simulink model "wecModel_Morrison_Heave_091514"  (R2014a)
settings: Solver=ode4  StartTime=0  StopTime=200  FixedStep=0.05  RelTol=1e-3
undefined symbols (not defined in the file): body, constraint, simu, waves, X, Y, Z
libraries: nesl_utility x18, vrlib x8, sm_lib x7, WECSim_Lib x2
(part 1 of 2)
settings Model: Creator=mlawson  LastModifiedBy=ntom
settings SolverCC: AlgebraicLoopSolver=LineSearch
settings DataIOCC: LimitDataPoints=off  SaveOutput=off  SaveTime=off
settings DebuggingCC: UnderspecifiedInitializationDetection=Classic  StateNameClashWarn=warning
settings ExplorerConfigSet: InternalSimMechanicsExplorerSettings="<ExplorerConfiguration><canonicalview>default</canonicalview><TilePanel><TileInfo><Tiles Columns=\"1\" Count=\"1\" Rows=\"1\"><Column Left=\"2\" Weight=\"1\"/><Column Left=\"1335\"/><Row Top=\"2\" Weight=\"1\"/><Row Top=\"911\"/><Tile Height=\"1\" Width=\"1\" X=\"0\" Y=\"0\"/></Tiles></TileInfo><SceneInfo><SceneViewer><BGColor><R>0.60000002384185791</R><G>0.60000002384185791</G><B>0.60000002384185791</B></BGColor><Camera><Position><X>365.37645888990272</X><Y>-369.82486814446582</Y><Z>359.64809521743916</Z></Position><Center><X>-6.7351450971904585</X><Y>2.2867358426280204</Y><Z>-12.463508769654169</Z></Center><Up><X>-0.40824829046386307</X><Y>0.40824829046386307</Y><Z>0.81649658092772615</Z></Up><Left>-57.820127362122818</Left><Right>57.820127362122818</Right><Bottom>-38.308817187253304</Bottom><Top>38.308817187253304</Top></Camera></SceneViewer></SceneInfo></TilePanel></ExplorerConfiguration>"

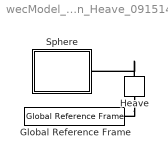
== system wecModel_Morrison_Heave_091514 ==
  Global Reference Frame : WECSim_Lib/Frames/Global Reference Frame  waves=waves  simu=simu
  Heave : WECSim_Lib/Constraints/Heave  constraint=constraint(1)
      settings: AttributesFormatString=%<constraint>
  Sphere : Subsystem  AncestorBlock=WECSim_Lib/Body Elements/Rigid Body  mask(BodyElements){body=body(1)}
      mask prompts: body "Body Name:"
      mask help: This block represents a rigid body. The variable name input below must be 'body(i)' where i=1,2,...
      mask init:
      | if exist('body','var')
      |     h=[gcb '/Structure/Body Properties'];
      |     geomFile=body.geom.file;
      |     set_param(h,'ExtGeomFileName',geomFile);
      |     h=[gcb '/To Workspace'];
      |     responseName=[body.name '_out'];
      |     set_param(h,'VariableName',responseName);
      | end
      | clear bc h geomFile responseName
      settings: AttributesFormatString=%<body>
  connections:
  Heave/RConn1 -- Sphere/RConn1
  Heave/LConn1 -- Global Reference Frame/RConn1

== system wecModel_Morrison_Heave_091514/Sphere ==
  Bus Creator : BusCreator  Inputs=5
  Bus Creator1 : BusCreator  Inputs=3
  Bus Selector : BusSelector  OutputSignals=disp,vel,accel
  Bus Selector1 : BusSelector  OutputSignals=F_Excitation,F_Restoring,F_Viscous,F_Mooring,F_Radiation
  Hydrostatic Restoring Force Calculation : Subsystem
  Mooring Force Calculation (Map) : Subsystem
  Structure : Subsystem
  Sum : Sum  Inputs=+----
  To Workspace : ToWorkspace  VariableName=Sphere_out  SaveFormat=Structure With Time  SampleTime=-1
  ViscousDampingForceCalculation : Subsystem
  Wave Diffraction and Excitation Force Calculation : Subsystem
  Wave Radiation Forces Calculation : Subsystem
  Conn : PMIOPort  Port=1  Side=Right
  wires:
  Bus Selector1/5 -> Sum/5  "<F_Radiation>"
  Bus Selector1/4 -> Sum/4  "<F_Mooring>"
  Bus Selector1/3 -> Sum/3  "<F_Viscous>"
  Bus Selector1/2 -> Sum/2  "<F_Restoring>"
  Bus Selector1/1 -> Sum/1  "<F_Excitation>"
  Wave Diffraction and Excitation Force Calculation/1(F_Excitation) -> Bus Creator/1
  Wave Radiation Forces Calculation/1(F_Radiation) -> Bus Creator/2
  Hydrostatic Restoring Force Calculation/1(F_Restoring) -> Bus Creator/3
  ViscousDampingForceCalculation/1(F_Viscous) -> Bus Creator/4
  Mooring Force Calculation (Map)/1(F_Mooring) -> Bus Creator/5
  Bus Selector/3 -> ViscousDampingForceCalculation/3(Acceleration), Wave Radiation Forces Calculation/2(Acceleration)  "<accel>"
  Bus Creator1/1 -> To Workspace/1
  Bus Creator/1 -> Bus Selector1/1, Bus Creator1/3
  Structure/1(Response) -> Bus Creator1/1, Bus Selector/1
  Bus Selector/2 -> Wave Radiation Forces Calculation/1(Velocity), Mooring Force Calculation (Map)/2(Velocity), ViscousDampingForceCalculation/1(Velocity)  "<vel>"
  Bus Selector/1 -> Hydrostatic Restoring Force Calculation/1(Displacement), Mooring Force Calculation (Map)/1(Displacement), ViscousDampingForceCalculation/2(Displacement)  "<disp>"
  Sum/1 -> Structure/1(F_vector), Bus Creator1/2
  connections:
  Structure/RConn1 -- Conn/RConn1

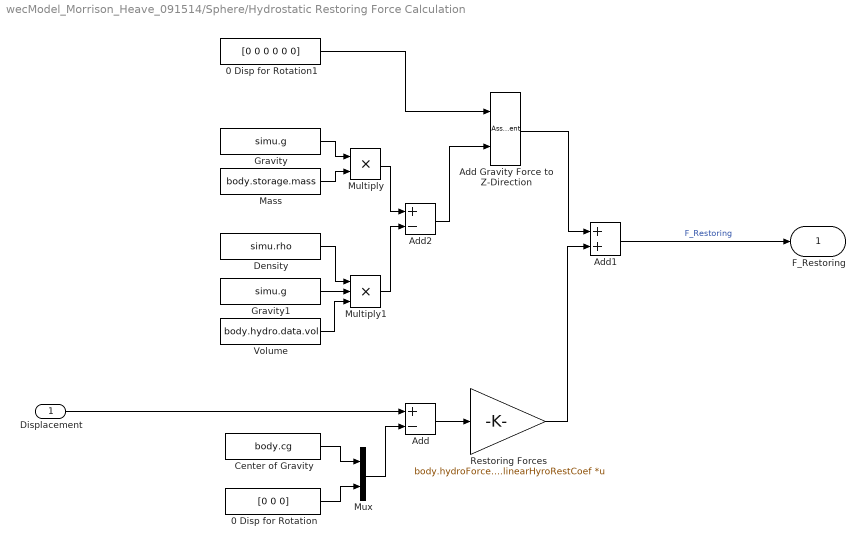
== system wecModel_Morrison_Heave_091514/Sphere/Hydrostatic Restoring Force Calculation ==
  Displacement : Inport
  0 Disp for Rotation : Constant  Value=[0 0 0]
  0 Disp for Rotation1 : Constant  Value=[0 0 0 0 0 0]
  Add : Sum  Inputs=+-
  Add Gravity Force to Z-Direction : Assignment  Indices=3
  Add1 : Sum
  Add2 : Sum  Inputs=+-
  Center of Gravity : Constant  Value=body.cg
  Density : Constant  Value=simu.rho
  Gravity : Constant  Value=simu.g
  Gravity1 : Constant  Value=simu.g
  Mass : Constant  Value=body.storage.mass
  Multiply : Product  Inputs=**
  Multiply1 : Product  Inputs=***
  Mux : Mux  Inputs=2
  Restoring Forces : Gain  Gain=body.hydroForce.linearHyroRestCoef  Multiplication=Matrix(K*u)
  Volume : Constant  Value=body.hydro.data.vol
  F_Restoring : Outport
  wires:
  Restoring Forces/1 -> Add1/2
  Add2/1 -> Add Gravity Force to Z-Direction/2
  Multiply1/1 -> Add2/2
  Multiply/1 -> Add2/1
  Density/1 -> Multiply1/1
  Gravity1/1 -> Multiply1/2
  Volume/1 -> Multiply1/3
  Add1/1 -> F_Restoring/1  "F_Restoring"
  Add Gravity Force to Z-Direction/1 -> Add1/1
  0 Disp for Rotation1/1 -> Add Gravity Force to Z-Direction/1
  Mass/1 -> Multiply/2
  Gravity/1 -> Multiply/1
  0 Disp for Rotation/1 -> Mux/2
  Center of Gravity/1 -> Mux/1
  Mux/1 -> Add/2
  Displacement/1 -> Add/1
  Add/1 -> Restoring Forces/1

== system wecModel_Morrison_Heave_091514/Sphere/Mooring Force Calculation (Map) ==
  Displacement : Inport
  Velocity : Inport  Port=2
  0 Disp for Rotation : Constant  Value=[0 0 0]
  Add : Sum  Inputs=+-
  Center of Gravity : Constant  Value=body.cg
  Mooring Damping : Gain  Gain=body.mooring.c  Multiplication=Matrix(K*u)
  Mooring Stiffness : Gain  Gain=body.mooring.k  Multiplication=Matrix(K*u)
  Mooring Pre-Tension : Constant  Value=body.mooring.preTension
  Mux : Mux  Inputs=2
  sum : Sum  Inputs=++-
  F_Mooring : Outport
  wires:
  0 Disp for Rotation/1 -> Mux/2
  Center of Gravity/1 -> Mux/1
  Displacement/1 -> Add/1
  Mux/1 -> Add/2
  Add/1 -> Mooring Stiffness/1
  Mooring Pre-Tension/1 -> sum/3
  sum/1 -> F_Mooring/1  "F_Mooring"
  Mooring Damping/1 -> sum/2
  Velocity/1 -> Mooring Damping/1
  Mooring Stiffness/1 -> sum/1

== system wecModel_Morrison_Heave_091514/Sphere/Structure ==
  F_vector : Inport
  Body CG : sm_lib/Frames and Transforms/Reference Frame  BlockFunction=simmechanics.library.frames_transforms.reference_frame
  Body Properties : sm_lib/Body Elements/Solid  InertiaType=Custom  Mass=body.mass  MassUnits=kg  CenterOfMass=[0 0 0]  CenterOfMassUnits=m  MomentsOfInertia=body.momOfInertia  MomentsOfInertiaUnits=kg*m^2  ProductsOfInertia=[0 0 0]  ProductsOfInertiaUnits=kg*m^2  DensityBased=on  Density=1000  DensityUnits=kg/(m^3)  GraphicType=FromGeometry  MarkerShape=Sphere  MarkerSize=10  MarkerSizeUnits=m  GraphicVisPropType=SimpleVisualProperties  GraphicDiffuseColor=[1 1 0]  GraphicSpecularColor=[0.5 0.5 0.5 1.0]  GraphicAmbientColor=[0.15 0.15 0.15 1.0]  GraphicEmissiveColor=[0.0 0.0 0.0 1.0]  GraphicShininess=75  GraphicOpacity=1  GeometryShape=FromFile  RectangleSize=[1 1]  RectangleSizeUnits=m  BrickDimensions=[1 1 1]  BrickDimensionUnits=m  CylinderRadius=1  CylinderRadiusUnits=m  CylinderLength=1  CylinderLengthUnits=m  SphereRadius=1  SphereRadiusUnits=m  EllipsoidRadii=[1 1 1]  EllipsoidRadiiUnits=m  ExtrusionCrossSection=[1 1; -1 1; -1 -1; 1 -1]  ExtrusionCrossSectionUnits=m  ExtrusionLength=1  ExtrusionLengthUnits=m  PolygonNumSides=3  PolygonOuterRadius=1  PolygonOuterRadiusUnits=m  ExtGeomFileType=STL  ExtGeomFileName=geometry/skewed_p4scaleZ_sphere_2m_neutral.stl  ExtGeomFileUnits=m  RevolutionCrossSection=[1 1; 1 -1; 2 -1; 2 1]  RevolutionCrossSectionUnits=m  RevolutionExtent=Full  RevolutionAngle=180  RevolutionAngleUnits=deg  BlockFunction=simmechanics.library.body_elements.solid
  Bus Creator : BusCreator  Inputs=3
  External Force and Torque : sm_lib/Forces and Torques/External Force and Torque  ForceResolutionFrame=World  EnableForceX=off  EnableForceY=off  EnableForceZ=off  EnableForce=on  TorqueResolutionFrame=World  EnableTorqueX=off  EnableTorqueY=off  EnableTorqueZ=off  EnableTorque=on  BlockFunction=simmechanics.library.forces_torques.external_force_torque
  Motion Sensor: Stucture Response : Subsystem
  Selector : Selector  InputPortWidth=6  Indices=[1:3]
  Selector1 : Selector  InputPortWidth=6  Indices=[4:6]
  Setup CG : sm_lib/Frames and Transforms/Rigid Transform  TranslationMethod=Cartesian  TranslationLengthUnit=m  TranslationStandardAxis=+Z  TranslationStandardOffset=0  TranslationCartesianOffset=body.cg  TranslationROffset=0  TranslationROffsetUnits=m  TranslationZOffset=0  TranslationZOffsetUnits=m  TranslationThetaOffset=0  TranslationThetaOffsetUnits=deg  RotationMethod=None  RotationAngleUnits=rad  RotationStandardAxis=+Y  RotationAngle=0.05  RotationArbitraryAxis=[0.57735026918962584 0.57735026918962584 0.57735026918962584]  FollAlignAxisA=+X  BaseAlignAxisA=+Y  FollAlignAxisB=+Y  BaseAlignAxisB=+Z  BlockFunction=simmechanics.library.frames_transforms.rigid_transform
  Setup Initial Disp : sm_lib/Frames and Transforms/Rigid Transform  TranslationMethod=Cartesian  TranslationLengthUnit=m  TranslationStandardAxis=+Z  TranslationStandardOffset=0  TranslationCartesianOffset=body.initLinDisp  TranslationROffset=0  TranslationROffsetUnits=m  TranslationZOffset=0  TranslationZOffsetUnits=m  TranslationThetaOffset=0  TranslationThetaOffsetUnits=deg  RotationMethod=ArbitraryAxis  RotationAngleUnits=rad  RotationStandardAxis=+Y  RotationAngle=body.initAngularDispAngle  RotationArbitraryAxis=body.initAngularDispAxis  FollAlignAxisA=+X  BaseAlignAxisA=+Y  FollAlignAxisB=+Y  BaseAlignAxisB=+Z  BlockFunction=simmechanics.library.frames_transforms.rigid_transform
  Simulink-PS Converter1 : nesl_utility/Simulink-PS Converter  PhysicalDomain=network_engine_domain  SubClassName=ps_input  LeftPortType=input  RightPortType=output  PseudoPeriodic=off  Frequencies=[]  NoiseDistribution=none  NoiseParameters=[]  Unit=1  AffineConversion=off  InputFiltering=off  SimscapeFilterOrder=1  InputFilterTimeConstant=0.001  UdotUserProvided=1
  Simulink-PS Converter2 : nesl_utility/Simulink-PS Converter  PhysicalDomain=network_engine_domain  SubClassName=ps_input  LeftPortType=input  RightPortType=output  PseudoPeriodic=off  Frequencies=[]  NoiseDistribution=none  NoiseParameters=[]  Unit=1  AffineConversion=off  InputFiltering=off  SimscapeFilterOrder=1  InputFilterTimeConstant=0.001  UdotUserProvided=1
  World Frame : sm_lib/Frames and Transforms/World Frame  BlockFunction=simmechanics.library.frames_transforms.world_frame
  Connection(MFS) : PMIOPort  Port=1  Side=Right
  Response : Outport
  wires:
  Motion Sensor: Stucture Response/3(Acceleration) -> Bus Creator/3  "accel"
  Motion Sensor: Stucture Response/2(Velocity) -> Bus Creator/2  "vel"
  Motion Sensor: Stucture Response/1(Displacement) -> Bus Creator/1  "disp"
  Bus Creator/1 -> Response/1  "response"
  Selector1/1 -> Simulink-PS Converter2/1
  Selector/1 -> Simulink-PS Converter1/1
  F_vector/1 -> Selector/1, Selector1/1
  connections:
  Motion Sensor: Stucture Response/RConn1 -- Body CG/RConn1 -- External Force and Torque/RConn1 -- Body Properties/RConn1 -- Setup Initial Disp/RConn1
  World Frame/RConn1 -- Motion Sensor: Stucture Response/LConn1
  Setup Initial Disp/LConn1 -- Setup CG/RConn1
  Setup CG/LConn1 -- Connection(MFS)/RConn1
  Simulink-PS Converter2/RConn1 -- External Force and Torque/LConn2
  Simulink-PS Converter1/RConn1 -- External Force and Torque/LConn1

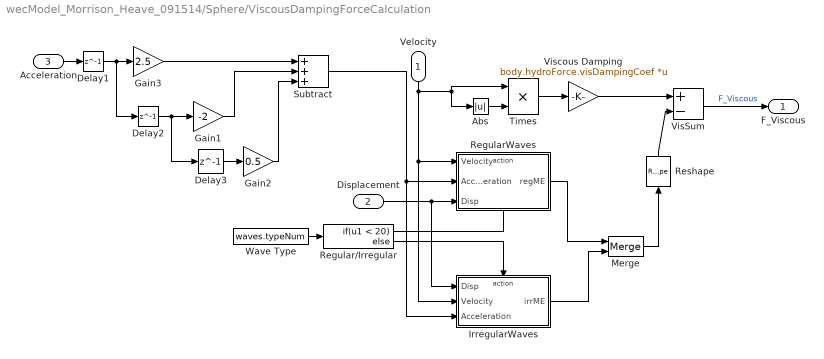
== system wecModel_Morrison_Heave_091514/Sphere/ViscousDampingForceCalculation ==
  Velocity : Inport
  Displacement : Inport  Port=2
  Acceleration : Inport  Port=3
  Abs : Abs
  Delay1 : Delay  DelayLength=1  InitialCondition=0
  Delay2 : Delay  DelayLength=1  InitialCondition=0
  Delay3 : Delay  DelayLength=1  InitialCondition=0
  Gain1 : Gain  Gain=-2
  Gain2 : Gain  Gain=0.5
  Gain3 : Gain  Gain=2.5
  IrregularWaves : Subsystem  TreatAsAtomicUnit=on
  Merge : Merge
  Regular/Irregular : If  IfExpression=u1 < 20
  RegularWaves : Subsystem  TreatAsAtomicUnit=on
  Reshape : Reshape
  Subtract : Sum  Inputs=+++
  Times : Product  Inputs=**
  "VisSum " : Sum  Inputs=+-
  Viscous Damping : Gain  Gain=body.hydroForce.visDampingCoef  Multiplication=Matrix(K*u)
  Wave Type : Constant  Value=waves.typeNum
  F_Viscous : Outport
  wires:
  Times/1 -> Viscous Damping/1
  Abs/1 -> Times/2
  Velocity/1 -> IrregularWaves/2(Velocity), RegularWaves/1(Velocity), Times/1, Abs/1
  Viscous Damping/1 -> "VisSum "/1
  "VisSum "/1 -> F_Viscous/1  "F_Viscous"
  Reshape/1 -> "VisSum "/2
  Wave Type/1 -> Regular/Irregular/1
  Regular/Irregular/2 -> IrregularWaves/Action
  Displacement/1 -> IrregularWaves/1(Disp), RegularWaves/3(Disp)
  Subtract/1 -> IrregularWaves/3(Acceleration), RegularWaves/2(Acceleration)
  Regular/Irregular/1 -> RegularWaves/Action
  IrregularWaves/1(irrME) -> Merge/2
  RegularWaves/1(regME) -> Merge/1
  Merge/1 -> Reshape/1
  Acceleration/1 -> Delay1/1
  Gain2/1 -> Subtract/3
  Gain1/1 -> Subtract/2
  Delay3/1 -> Gain2/1
  Delay2/1 -> Gain1/1, Delay3/1
  Delay1/1 -> Delay2/1, Gain3/1
  Gain3/1 -> Subtract/1

== system wecModel_Morrison_Heave_091514/Sphere/Wave Diffraction and Excitation Force Calculation ==
  Applied Ramp Function : Subsystem  TreatAsAtomicUnit=on
  If : If  IfExpression=u1 < 20
  If1 : If  NumInputs=2  IfExpression=u1 < u2
  Iregular Wave Excitation Force : Subsystem  TreatAsAtomicUnit=on
  Merge : Merge
  Merge1 : Merge
  No Ramp Function : Subsystem  TreatAsAtomicUnit=on
  Ramp Function Time : Constant  Value=simu.rampT
  Regular Wave Excitation Force : Subsystem  TreatAsAtomicUnit=on
  Wave Type : Constant  Value=waves.typeNum
  F_Excitation : Outport
  wires:
  Wave Type/1 -> If/1
  If/1 -> Regular Wave Excitation Force/Action
  If/2 -> Iregular Wave Excitation Force/Action
  Regular Wave Excitation Force/1(F_wave) -> Merge/1
  Iregular Wave Excitation Force/1(F_wave) -> Merge/2
  Ramp Function Time/1 -> If1/2
  Merge/1 -> No Ramp Function/1(In1), Applied Ramp Function/1(In1)
  If1/2 -> No Ramp Function/Action
  If1/1 -> Applied Ramp Function/Action
  Applied Ramp Function/1(Out1) -> Merge1/1
  No Ramp Function/1(Out1) -> Merge1/2
  Merge1/1 -> F_Excitation/1  "F_Excitation"
  [Clock] -> If1/1, Iregular Wave Excitation Force/1(Time)

== system wecModel_Morrison_Heave_091514/Sphere/Wave Radiation Forces Calculation ==
  Velocity : Inport
  Acceleration : Inport  Port=2
  Added Mass Forces : Gain  Gain=body.hydroForce.fAddedMass  Multiplication=Matrix(K*u)
  Damping Forces : Gain  Gain=body.hydroForce.fDamping  Multiplication=Matrix(K*u)
  Delay : Delay  DelayLength=1  InitialCondition=0
  Delay1 : Delay  DelayLength=1  InitialCondition=0
  Delay2 : Delay  DelayLength=1  InitialCondition=0
  Fluid Memory : MATLAB Function  TreatAsAtomicUnit=on
  Gain : Gain  Gain=2.5
  Gain1 : Gain  Gain=-2
  Gain2 : Gain  Gain=0.5
  Impulse Response Function K : Constant  Value=body.hydroForce.irkb
  Initial Zero Velocity : Constant  Value=simu.zeroVel
  Subtract : Sum  Inputs=+++
  Sum of Elements : Sum  Inputs=+++
  Time (relative to the current time step) : Constant  Value=simu.CTTime
  Wave Type : Constant  Value=waves.typeNum
  F_Radiation : Outport
  wires:
  Sum of Elements/1 -> F_Radiation/1  "F_Radiation"
  Gain2/1 -> Subtract/3
  Gain1/1 -> Subtract/2
  Delay2/1 -> Gain2/1
  Subtract/1 -> Added Mass Forces/1
  Delay1/1 -> Delay2/1, Gain1/1
  Gain/1 -> Subtract/1
  Delay/1 -> Gain/1, Delay1/1
  Acceleration/1 -> Delay/1
  Wave Type/1 -> Fluid Memory/1(check)
  Time (relative to the current time step)/1 -> Fluid Memory/5(CTTime)
  Impulse Response Function K/1 -> Fluid Memory/4(IRKB)
  Initial Zero Velocity/1 -> Fluid Memory/3(ZeroVel)
  Velocity/1 -> Damping Forces/1, Fluid Memory/2(v)
  Damping Forces/1 -> Sum of Elements/1  "F_Radiation Damping"
  Added Mass Forces/1 -> Sum of Elements/3  "F_Added Mass"
  Fluid Memory/1(F_FM) -> Sum of Elements/2  "F_Convolution Integral"

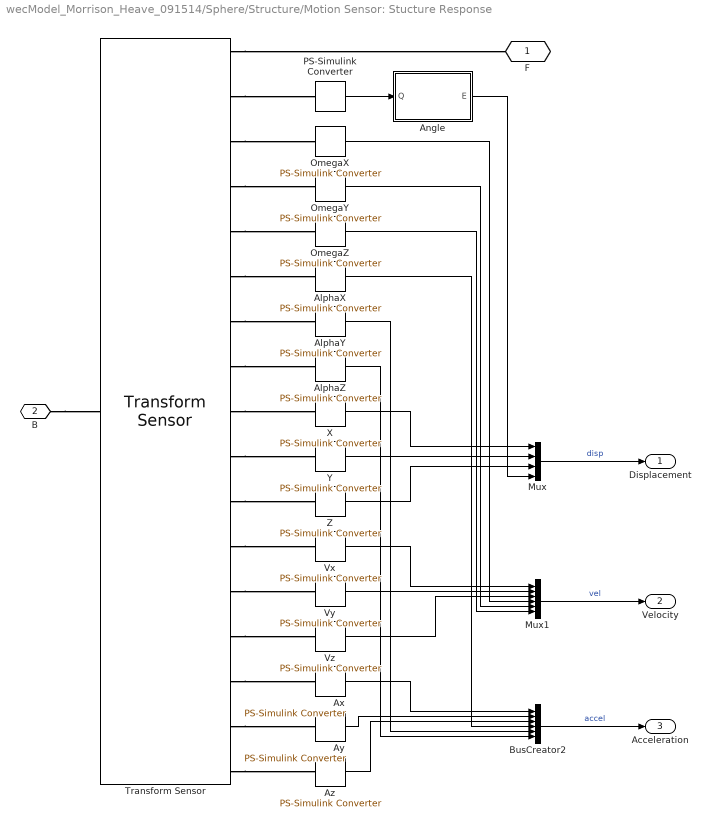
== system wecModel_Morrison_Heave_091514/Sphere/Structure/Motion Sensor: Stucture Response ==
  AlphaX : nesl_utility/PS-Simulink Converter  PhysicalDomain=network_engine_domain  SubClassName=ps_output  LeftPortType=input  RightPortType=output  PseudoPeriodic=off  Frequencies=[]  Unit=1  AffineConversion=off
  "AlphaY " : nesl_utility/PS-Simulink Converter  PhysicalDomain=network_engine_domain  SubClassName=ps_output  LeftPortType=input  RightPortType=output  PseudoPeriodic=off  Frequencies=[]  Unit=1  AffineConversion=off
  AlphaZ : nesl_utility/PS-Simulink Converter  PhysicalDomain=network_engine_domain  SubClassName=ps_output  LeftPortType=input  RightPortType=output  PseudoPeriodic=off  Frequencies=[]  Unit=1  AffineConversion=off
  Angle : MATLAB Function  TreatAsAtomicUnit=on
  Ax : nesl_utility/PS-Simulink Converter  PhysicalDomain=network_engine_domain  SubClassName=ps_output  LeftPortType=input  RightPortType=output  PseudoPeriodic=off  Frequencies=[]  Unit=1  AffineConversion=off
  Ay : nesl_utility/PS-Simulink Converter  PhysicalDomain=network_engine_domain  SubClassName=ps_output  LeftPortType=input  RightPortType=output  PseudoPeriodic=off  Frequencies=[]  Unit=1  AffineConversion=off
  Az : nesl_utility/PS-Simulink Converter  PhysicalDomain=network_engine_domain  SubClassName=ps_output  LeftPortType=input  RightPortType=output  PseudoPeriodic=off  Frequencies=[]  Unit=1  AffineConversion=off
  BusCreator2 : BusCreator  Inputs=6
  Mux : Mux
  Mux1 : Mux  Inputs=6
  OmegaX : nesl_utility/PS-Simulink Converter  PhysicalDomain=network_engine_domain  SubClassName=ps_output  LeftPortType=input  RightPortType=output  PseudoPeriodic=off  Frequencies=[]  Unit=1  AffineConversion=off
  OmegaY : nesl_utility/PS-Simulink Converter  PhysicalDomain=network_engine_domain  SubClassName=ps_output  LeftPortType=input  RightPortType=output  PseudoPeriodic=off  Frequencies=[]  Unit=1  AffineConversion=off
  OmegaZ : nesl_utility/PS-Simulink Converter  PhysicalDomain=network_engine_domain  SubClassName=ps_output  LeftPortType=input  RightPortType=output  PseudoPeriodic=off  Frequencies=[]  Unit=1  AffineConversion=off
  PS-Simulink Converter : nesl_utility/PS-Simulink Converter  PhysicalDomain=network_engine_domain  SubClassName=ps_output  LeftPortType=input  RightPortType=output  PseudoPeriodic=off  Frequencies=[]  Unit=1  AffineConversion=off
  Transform Sensor : sm_lib/Frames and Transforms/Transform Sensor  MeasurementFrame=World  SenseAngle=off  SenseAxis=off  SenseAngle1=off  SenseAngle2=off  SenseAngle3=off  SenseQ=on  SenseR=off  SenseOmegaX=on  SenseOmegaY=on  SenseOmegaZ=on  SenseOmega1=off  SenseOmega2=off  SenseOmega3=off  SenseQDot=off  SenseRDot=off  SenseAlphaX=on  SenseAlphaY=on  SenseAlphaZ=on  SenseAlpha1=off  SenseAlpha2=off  SenseAlpha3=off  SenseQDDot=off  SenseRDDot=off  SenseX=on  SenseY=on  SenseZ=on  SenseRad=off  SenseAzim=off  SenseDist=off  SenseInc=off  SenseXDot=on  SenseYDot=on  SenseZDot=on  SenseRadDot=off  SenseAzimDot=off  SenseDistDot=off  SenseIncDot=off  SenseXDDot=on  SenseYDDot=on  SenseZDDot=on  SenseRadDDot=off  SenseAzimDDot=off  SenseDistDDot=off  SenseIncDDot=off  BlockFunction=simmechanics.library.frames_transforms.transform_sensor
  Vx : nesl_utility/PS-Simulink Converter  PhysicalDomain=network_engine_domain  SubClassName=ps_output  LeftPortType=input  RightPortType=output  PseudoPeriodic=off  Frequencies=[]  Unit=1  AffineConversion=off
  Vy : nesl_utility/PS-Simulink Converter  PhysicalDomain=network_engine_domain  SubClassName=ps_output  LeftPortType=input  RightPortType=output  PseudoPeriodic=off  Frequencies=[]  Unit=1  AffineConversion=off
  Vz : nesl_utility/PS-Simulink Converter  PhysicalDomain=network_engine_domain  SubClassName=ps_output  LeftPortType=input  RightPortType=output  PseudoPeriodic=off  Frequencies=[]  Unit=1  AffineConversion=off
  X : nesl_utility/PS-Simulink Converter  PhysicalDomain=network_engine_domain  SubClassName=ps_output  LeftPortType=input  RightPortType=output  PseudoPeriodic=off  Frequencies=[]  Unit=1  AffineConversion=off
  Y : nesl_utility/PS-Simulink Converter  PhysicalDomain=network_engine_domain  SubClassName=ps_output  LeftPortType=input  RightPortType=output  PseudoPeriodic=off  Frequencies=[]  Unit=1  AffineConversion=off
  Z : nesl_utility/PS-Simulink Converter  PhysicalDomain=network_engine_domain  SubClassName=ps_output  LeftPortType=input  RightPortType=output  PseudoPeriodic=off  Frequencies=[]  Unit=1  AffineConversion=off
  F : PMIOPort  Port=1  Side=Right
  B : PMIOPort  Port=2  Side=Left
  Displacement : Outport
  Velocity : Outport  Port=2
  Acceleration : Outport  Port=3
  wires:
  OmegaZ/1 -> Mux1/6
  OmegaY/1 -> Mux1/5
  OmegaX/1 -> Mux1/4
  AlphaZ/1 -> BusCreator2/6
  "AlphaY "/1 -> BusCreator2/5
  Z/1 -> Mux/3
  Y/1 -> Mux/2
  X/1 -> Mux/1
  Angle/1(E) -> Mux/4
  BusCreator2/1 -> Acceleration/1  "accel"
  Mux1/1 -> Velocity/1  "vel"
  Mux/1 -> Displacement/1  "disp"
  Az/1 -> BusCreator2/3
  Ay/1 -> BusCreator2/2
  Ax/1 -> BusCreator2/1
  Vz/1 -> Mux1/3
  Vy/1 -> Mux1/2
  Vx/1 -> Mux1/1
  AlphaX/1 -> BusCreator2/4
  PS-Simulink Converter/1 -> Angle/1(Q)
  connections:
  Transform Sensor/RConn5 -- OmegaZ/LConn1
  Transform Sensor/RConn4 -- OmegaY/LConn1
  Transform Sensor/RConn3 -- OmegaX/LConn1
  Transform Sensor/RConn8 -- AlphaZ/LConn1
  Transform Sensor/RConn7 -- "AlphaY "/LConn1
  Transform Sensor/RConn6 -- AlphaX/LConn1
  Transform Sensor/RConn9 -- X/LConn1
  Transform Sensor/RConn10 -- Y/LConn1
  Transform Sensor/RConn11 -- Z/LConn1
  Transform Sensor/RConn12 -- Vx/LConn1
  Transform Sensor/RConn13 -- Vy/LConn1
  Transform Sensor/RConn14 -- Vz/LConn1
  Transform Sensor/RConn15 -- Ax/LConn1
  Transform Sensor/RConn16 -- Ay/LConn1
  Transform Sensor/RConn17 -- Az/LConn1
  Transform Sensor/RConn2 -- PS-Simulink Converter/LConn1
  B/RConn1 -- Transform Sensor/LConn1
  Transform Sensor/RConn1 -- F/RConn1

== system wecModel_Morrison_Heave_091514/Sphere/ViscousDampingForceCalculation/IrregularWaves ==
  Disp : Inport
  Velocity : Inport  Port=2
  Acceleration : Inport  Port=3
  Action Port : ActionPort
  Area : Constant  Value=body.characteristicAreaME  VectorParams1D=off
  Ca : Constant  Value=body.Ca  VectorParams1D=off
  Cd : Constant  Value=body.cdME  VectorParams1D=off
  MESum : Sum  Inputs=+  CollapseMode=Specified dimension
  MorrisonElements : Subsystem  TreatAsAtomicUnit=on
  Volume : Constant  Value=body.VME  VectorParams1D=off
  "r_{g}" : Constant  Value=body.rgME  VectorParams1D=off
  irrME : Outport
  wires:
  Velocity/1 -> MorrisonElements/2(Vel)
  "r_{g}"/1 -> MorrisonElements/1(r)
  Area/1 -> MorrisonElements/5(A)
  Cd/1 -> MorrisonElements/6(Cd)
  Disp/1 -> MorrisonElements/4(Disp)
  Acceleration/1 -> MorrisonElements/3(Accel)
  Volume/1 -> MorrisonElements/7(Vol)
  Ca/1 -> MorrisonElements/8(Ca)
  MorrisonElements/1(Force) -> MESum/1
  MESum/1 -> irrME/1

== system wecModel_Morrison_Heave_091514/Sphere/ViscousDampingForceCalculation/RegularWaves ==
  Velocity : Inport
  Acceleration : Inport  Port=2
  Disp : Inport  Port=3
  Action Port : ActionPort
  Area : Constant  Value=body.characteristicAreaME  VectorParams1D=off
  Ca : Constant  Value=body.Ca  VectorParams1D=off
  Cd : Constant  Value=body.cdME  VectorParams1D=off
  MESum : Sum  Inputs=+  CollapseMode=Specified dimension
  MorrisonElements : Subsystem  TreatAsAtomicUnit=on
  Volume : Constant  Value=body.VME  VectorParams1D=off
  "r_{g}" : Constant  Value=body.rgME  VectorParams1D=off
  regME : Outport
  wires:
  MESum/1 -> regME/1
  Velocity/1 -> MorrisonElements/2(Vel)
  "r_{g}"/1 -> MorrisonElements/1(r)
  Area/1 -> MorrisonElements/5(A)
  Cd/1 -> MorrisonElements/6(Cd)
  Disp/1 -> MorrisonElements/4(Disp)
  Acceleration/1 -> MorrisonElements/3(Accel)
  MorrisonElements/1(Force) -> MESum/1
  Volume/1 -> MorrisonElements/7(Vol)
  Ca/1 -> MorrisonElements/8(Ca)

== system wecModel_Morrison_Heave_091514/Sphere/Wave Diffraction and Excitation Force Calculation/Applied Ramp Function ==
  In1 : Inport
  Action Port : ActionPort
  Add : Sum
  Constant : Constant  Value=2
  Constant1 : Constant
  Divide : Product  Inputs=**/
  Sine Wave : Sin  Frequency=pi/simu.rampT  Phase=pi+pi/2  SampleTime=0
  Out1 : Outport
  wires:
  In1/1 -> Divide/1
  Divide/1 -> Out1/1
  Constant/1 -> Divide/3
  Constant1/1 -> Add/1
  Sine Wave/1 -> Add/2
  Add/1 -> Divide/2

== system wecModel_Morrison_Heave_091514/Sphere/Wave Diffraction and Excitation Force Calculation/Iregular Wave Excitation Force ==
  Time : Inport
  Action Port : ActionPort
  Excitation Re Part2 : Constant  Value=body.hydroForce.fExt.re  VectorParams1D=off
  Excitation Re Part3 : Constant  Value=body.hydroForce.fExt.im  VectorParams1D=off
  For Each Subsystem : Subsystem  TreatAsAtomicUnit=on
  Sum of Elements : Sum  Inputs=+  CollapseMode=Specified dimension
  dw1 : Constant  Value=(waves.w(end)-waves.w(1))/(waves.numFreq-1)  VectorParams1D=off
  wave frequency : Constant  Value=waves.w  VectorParams1D=off
  wave frequency1 : Constant  Value=waves.phaseRand'  VectorParams1D=off
  wave spectrum : Constant  Value=waves.A*2  VectorParams1D=off
  F_wave : Outport  PortDimensions=6
  wires:
  Excitation Re Part2/1 -> For Each Subsystem/3(wave fExt re)
  Excitation Re Part3/1 -> For Each Subsystem/4(wave fExt im)
  wave frequency/1 -> For Each Subsystem/2(wave freq)
  wave spectrum/1 -> For Each Subsystem/1(wave spectrum)
  For Each Subsystem/1(Out1) -> Sum of Elements/1
  Time/1 -> For Each Subsystem/5(Time)
  Sum of Elements/1 -> F_wave/1
  wave frequency1/1 -> For Each Subsystem/7(phaseRand)
  dw1/1 -> For Each Subsystem/6(dw)

== system wecModel_Morrison_Heave_091514/Sphere/Wave Diffraction and Excitation Force Calculation/No Ramp Function ==
  In1 : Inport
  Action Port : ActionPort
  Out1 : Outport
  wires:
  In1/1 -> Out1/1

== system wecModel_Morrison_Heave_091514/Sphere/Wave Diffraction and Excitation Force Calculation/Regular Wave Excitation Force ==
  Action Port : ActionPort
  Add : Sum  Inputs=+-
  Cos Wave : Sin  Amplitude=waves.A(1,:)  Frequency=waves.w(1,:)  Phase=pi/2  SampleTime=0
  Product : Product  Inputs=**
  Product1 : Product  Inputs=**
  Sin Wave : Sin  Amplitude=waves.A(1,:)  Frequency=waves.w(1,:)  SampleTime=0
  WAMIT Excitation Im Part : Constant  Value=body.hydroForce.fExt.im(1,:)  VectorParams1D=off
  WAMIT Excitation Re Part : Constant  Value=body.hydroForce.fExt.re(1,:)  VectorParams1D=off
  F_wave : Outport  PortDimensions=6
  wires:
  Cos Wave/1 -> Product/1
  WAMIT Excitation Re Part/1 -> Product/2
  Sin Wave/1 -> Product1/1
  Product1/1 -> Add/2
  WAMIT Excitation Im Part/1 -> Product1/2
  Product/1 -> Add/1
  Add/1 -> F_wave/1

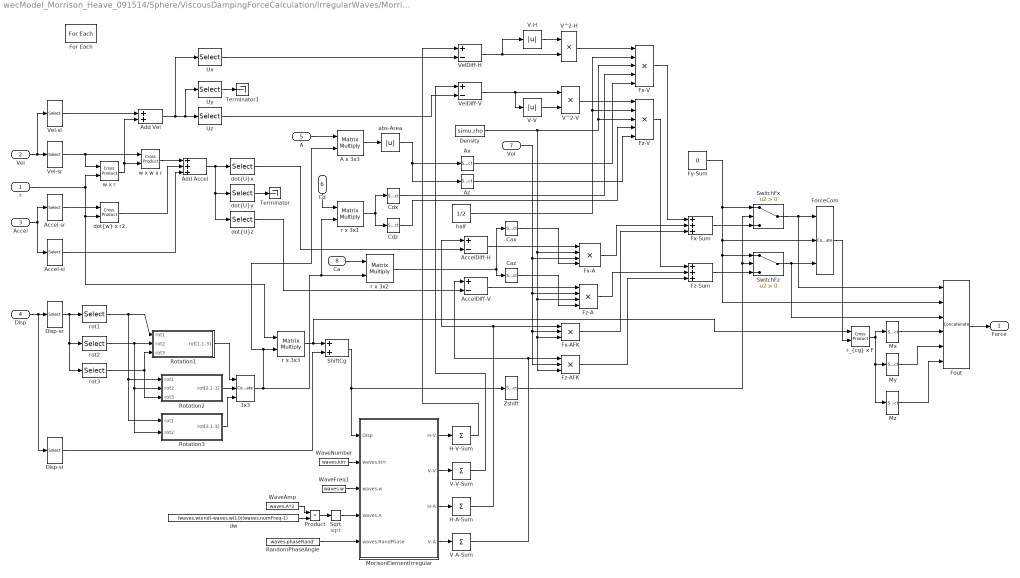
== system wecModel_Morrison_Heave_091514/Sphere/ViscousDampingForceCalculation/IrregularWaves/MorrisonElements ==
  r : Inport  Partition=on  PartitionDimension=1  PartitionWidth=1
  Vel : Inport  Port=2  Partition=off
  Accel : Inport  Port=3  Partition=off
  Disp : Inport  Port=4  Partition=off
  A : Inport  Port=5  Partition=on  PartitionDimension=1  PartitionWidth=1
  Cd : Inport  Port=6  Partition=on  PartitionDimension=1  PartitionWidth=1
  Vol : Inport  Port=7  Partition=on  PartitionDimension=1  PartitionWidth=1
  Ca : Inport  Port=8  Partition=on  PartitionDimension=1  PartitionWidth=1
  3x3 : Concatenate  NumInputs=3  Mode=Multidimensional array
  A x 3x3 : Product  Multiplication=Matrix(*)
  Accel-sl : Selector  InputPortWidth=6  Indices=[1 2 3]
  Accel-sr : Selector  InputPortWidth=6  Indices=[4 5 6]
  AccelDiff-H : Sum  Inputs=+-
  AccelDiff-V : Sum  Inputs=+-
  Add Accel : Sum  Inputs=+++
  Add Vel : Sum
  Ax : Selector  InputPortWidth=3  Indices=[1]
  Az : Selector  InputPortWidth=3  Indices=[3]
  Cax : Selector  InputPortWidth=3  Indices=[1]
  Caz : Selector  InputPortWidth=3  Indices=[3]
  Cdx : Selector  InputPortWidth=3  Indices=[1]
  Cdz : Selector  InputPortWidth=3  Indices=[3]
  Density : Constant  Value=simu.rho
  Disp-sl : Selector  InputPortWidth=6  Indices=[1 2 3]
  Disp-sr : Selector  InputPortWidth=6  Indices=[4 5 6]
  For Each : ForEach  DisableCoverage=on  IndexMode=One-based
  ForceCom : Concatenate  NumInputs=3  ConcatenateDimension=2
  Fout : Concatenate  NumInputs=6  Mode=Multidimensional array  ConcatenateDimension=2
  Fx-A : Product  Inputs=4
  Fx-AFK : Product  Inputs=3
  Fx-Sum : Sum  Inputs=+++
  Fx-V : Product  Inputs=5
  Fy-Sum : Constant  Value=0
  Fz-A : Product  Inputs=4
  Fz-AFK : Product  Inputs=3
  Fz-Sum : Sum  Inputs=+++
  Fz-V : Product  Inputs=5
  H-A-Sum : Sum  Inputs=+  CollapseMode=Specified dimension
  H-V-Sum : Sum  Inputs=+  CollapseMode=Specified dimension
  MorisonElementIrregular : Subsystem  TreatAsAtomicUnit=on
  Mx : Selector  InputPortWidth=3  Indices=[1]
  My : Selector  InputPortWidth=3  Indices=[2]
  Mz : Selector  InputPortWidth=3  Indices=[3]
  Product : Product
  RandomPhaseAngle : Constant  Value=waves.phaseRand'  VectorParams1D=off
  Rotation1 : Subsystem
  Rotation2 : Subsystem
  Rotation3 : Subsystem
  ShiftCg : Sum
  Sqrt : Sqrt  SaturateOnIntegerOverflow=on
  SwitchFx : Switch  Criteria=u2 > Threshold
  SwitchFz : Switch  Criteria=u2 > Threshold
  Terminator : Terminator
  Terminator1 : Terminator
  Ux : Selector  InputPortWidth=3  Indices=[1]
  Uy : Selector  InputPortWidth=3  Indices=[2]
  Uz : Selector  InputPortWidth=3  Indices=[3]
  V-A-Sum : Sum  Inputs=+  CollapseMode=Specified dimension
  V-H : Abs
  V-V : Abs
  V-V-Sum : Sum  Inputs=+  CollapseMode=Specified dimension
  V^2-H : Product
  V^2-V : Product
  Vel-sl : Selector  InputPortWidth=6  Indices=[1 2 3]
  "Vel-sr " : Selector  InputPortWidth=6  Indices=[4 5 6]
  VelDiff-H : Sum  Inputs=+-
  VelDiff-V : Sum  Inputs=+-
  WaveAmp : Constant  Value=waves.A*2  VectorParams1D=off
  WaveFreq1 : Constant  Value=waves.w  VectorParams1D=off
  WaveNumber : Constant  Value=waves.kirr  VectorParams1D=off
  Zshift : Selector  InputPortWidth=3  Indices=[3]
  abs-Area : Abs
  "dot{U}x" : Selector  InputPortWidth=3  Indices=[1]
  "dot{U}y" : Selector  InputPortWidth=3  Indices=[2]
  "dot{U}z" : Selector  InputPortWidth=3  Indices=[3]
  "dot{w} x r2" : vrlib/Utilities/Cross Product
  dw : Constant  Value=(waves.w(end)-waves.w(1))/(waves.numFreq-1)  VectorParams1D=off
  half : Constant  Value=1/2
  r x 3x1 : Product  Multiplication=Matrix(*)
  r x 3x2 : Product  Multiplication=Matrix(*)
  r x 3x3 : Product  Multiplication=Matrix(*)
  "r_{cg} x F" : vrlib/Utilities/Cross Product
  rot1 : Selector  InputPortWidth=3  Indices=[1]
  rot2 : Selector  InputPortWidth=3  Indices=[2]
  rot3 : Selector  InputPortWidth=3  Indices=[3]
  w x r : vrlib/Utilities/Cross Product
  w x w x r : vrlib/Utilities/Cross Product
  Force : Outport  PortDimensions=[1 6]  ConcatenationDimension=1
  wires:
  Vel/1 -> Vel-sl/1, "Vel-sr "/1
  w x r/1 -> Add Vel/2, w x w x r/2
  w x w x r/1 -> Add Accel/1
  "Vel-sr "/1 -> w x w x r/1, w x r/1
  r/1 -> r x 3x3/1, "dot{w} x r2"/2, w x r/2
  Accel/1 -> Accel-sl/1, Accel-sr/1
  Accel-sr/1 -> "dot{w} x r2"/1
  "dot{w} x r2"/1 -> Add Accel/2
  Accel-sl/1 -> Add Accel/3
  Add Accel/1 -> "dot{U}z"/1, "dot{U}y"/1, "dot{U}x"/1
  Vel-sl/1 -> Add Vel/1
  Disp/1 -> Disp-sl/1, Disp-sr/1
  Disp-sr/1 -> rot3/1, rot2/1, rot1/1
  rot3/1 -> Rotation2/3(rot3), Rotation1/3(rot3)
  rot1/1 -> Rotation3/1(rot1), Rotation2/1(rot1), Rotation1/1(rot1)
  rot2/1 -> Rotation3/2(rot2), Rotation2/2(rot2), Rotation1/2(rot2)
  Rotation2/1(rot[2,1-3]) -> 3x3/2
  Rotation1/1(rot[1,1-3]) -> 3x3/1
  Rotation3/1(rot[3,1-3]) -> 3x3/3
  r x 3x3/1 -> "r_{cg} x F"/1, ShiftCg/1
  Disp-sl/1 -> ShiftCg/2
  ShiftCg/1 -> MorisonElementIrregular/1(Disp), Zshift/1
  "dot{U}y"/1 -> Terminator/1
  "dot{U}x"/1 -> AccelDiff-H/2
  H-A-Sum/1 -> AccelDiff-H/1, Fx-AFK/1
  "dot{U}z"/1 -> AccelDiff-V/2
  Add Vel/1 -> Uy/1, Uz/1, Ux/1
  Uy/1 -> Terminator1/1
  Ux/1 -> VelDiff-H/2
  Uz/1 -> VelDiff-V/2
  H-V-Sum/1 -> VelDiff-H/1
  V-V-Sum/1 -> VelDiff-V/1
  V-V/1 -> V^2-V/2
  VelDiff-V/1 -> V-V/1, V^2-V/1
  V^2-H/1 -> Fx-V/1
  half/1 -> Fz-V/2, Fx-V/2
  Density/1 -> Fx-AFK/3, Fz-AFK/3, Fz-A/3, Fx-A/2, Fz-V/3, Fx-V/3
  V^2-V/1 -> Fz-V/1
  AccelDiff-H/1 -> Fx-A/1
  Vol/1 -> Fz-AFK/2, Fx-AFK/2, Fz-A/2, Fx-A/3
  AccelDiff-V/1 -> Fz-A/1
  V-A-Sum/1 -> AccelDiff-V/1, Fz-AFK/1
  Fx-V/1 -> Fx-Sum/1
  Fx-A/1 -> Fx-Sum/2
  Fx-AFK/1 -> Fx-Sum/3
  Fz-V/1 -> Fz-Sum/1
  Fz-A/1 -> Fz-Sum/2
  Fz-AFK/1 -> Fz-Sum/3
  Fy-Sum/1 -> SwitchFx/1, ForceCom/2, SwitchFz/1, Fout/2
  "r_{cg} x F"/1 -> Mz/1, My/1, Mx/1
  Mx/1 -> Fout/4
  My/1 -> Fout/5
  Mz/1 -> Fout/6
  3x3/1 -> A x 3x3/2, r x 3x3/2, r x 3x2/2, r x 3x1/2
  VelDiff-H/1 -> V-H/1, V^2-H/2
  Zshift/1 -> SwitchFz/2, SwitchFx/2
  SwitchFz/1 -> Fout/3, ForceCom/3
  SwitchFx/1 -> Fout/1, ForceCom/1
  Fx-Sum/1 -> SwitchFx/3
  Fz-Sum/1 -> SwitchFz/3
  Az/1 -> Fz-V/5
  A/1 -> A x 3x3/1
  Ax/1 -> Fx-V/5
  Cdx/1 -> Fx-V/4
  Cdz/1 -> Fz-V/4
  A x 3x3/1 -> abs-Area/1
  abs-Area/1 -> Az/1, Ax/1
  ForceCom/1 -> "r_{cg} x F"/2
  Fout/1 -> Force/1
  Caz/1 -> Fz-A/4
  Cax/1 -> Fx-A/4
  Cd/1 -> r x 3x1/1
  r x 3x1/1 -> Cdz/1, Cdx/1
  Ca/1 -> r x 3x2/1
  r x 3x2/1 -> Cax/1, Caz/1
  WaveNumber/1 -> MorisonElementIrregular/2(waves.kirr)
  WaveFreq1/1 -> MorisonElementIrregular/3(waves.w)
  RandomPhaseAngle/1 -> MorisonElementIrregular/5(waves.RandPhase)
  MorisonElementIrregular/1(H-V) -> H-V-Sum/1
  WaveAmp/1 -> Product/1
  dw/1 -> Product/2
  Product/1 -> Sqrt/1
  Sqrt/1 -> MorisonElementIrregular/4(waves.A)
  MorisonElementIrregular/2(V-V) -> V-V-Sum/1
  MorisonElementIrregular/3(H-A) -> H-A-Sum/1
  MorisonElementIrregular/4(V-A) -> V-A-Sum/1
  V-H/1 -> V^2-H/1

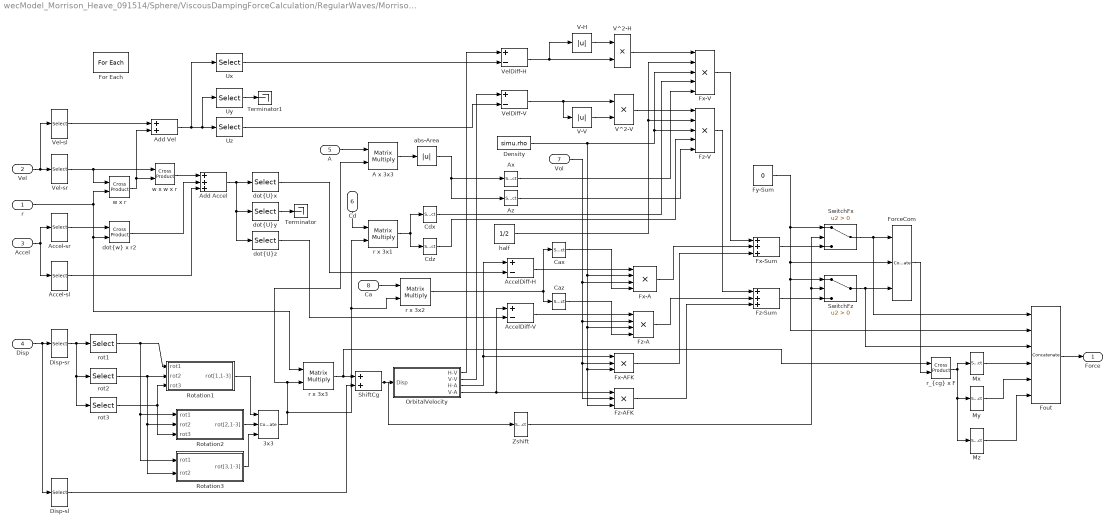
== system wecModel_Morrison_Heave_091514/Sphere/ViscousDampingForceCalculation/RegularWaves/MorrisonElements ==
  r : Inport  Partition=on  PartitionDimension=1  PartitionWidth=1
  Vel : Inport  Port=2  Partition=off
  Accel : Inport  Port=3  Partition=off
  Disp : Inport  Port=4  Partition=off
  A : Inport  Port=5  Partition=on  PartitionDimension=1  PartitionWidth=1
  Cd : Inport  Port=6  Partition=on  PartitionDimension=1  PartitionWidth=1
  Vol : Inport  Port=7  Partition=on  PartitionDimension=1  PartitionWidth=1
  Ca : Inport  Port=8  Partition=on  PartitionDimension=1  PartitionWidth=1
  3x3 : Concatenate  NumInputs=3  Mode=Multidimensional array
  A x 3x3 : Product  Multiplication=Matrix(*)
  Accel-sl : Selector  InputPortWidth=6  Indices=[1 2 3]
  Accel-sr : Selector  InputPortWidth=6  Indices=[4 5 6]
  AccelDiff-H : Sum  Inputs=+-
  AccelDiff-V : Sum  Inputs=+-
  Add Accel : Sum  Inputs=+++
  Add Vel : Sum
  Ax : Selector  InputPortWidth=3  Indices=[1]
  Az : Selector  InputPortWidth=3  Indices=[3]
  Cax : Selector  InputPortWidth=3  Indices=[1]
  Caz : Selector  InputPortWidth=3  Indices=[3]
  Cdx : Selector  InputPortWidth=3  Indices=[1]
  Cdz : Selector  InputPortWidth=3  Indices=[3]
  Density : Constant  Value=simu.rho
  Disp-sl : Selector  InputPortWidth=6  Indices=[1 2 3]
  Disp-sr : Selector  InputPortWidth=6  Indices=[4 5 6]
  For Each : ForEach  DisableCoverage=on  IndexMode=One-based
  ForceCom : Concatenate  NumInputs=3  ConcatenateDimension=2
  Fout : Concatenate  NumInputs=6  Mode=Multidimensional array  ConcatenateDimension=2
  Fx-A : Product  Inputs=4
  Fx-AFK : Product  Inputs=3
  Fx-Sum : Sum  Inputs=+++
  Fx-V : Product  Inputs=5
  Fy-Sum : Constant  Value=0
  Fz-A : Product  Inputs=4
  Fz-AFK : Product  Inputs=3
  Fz-Sum : Sum  Inputs=+++
  Fz-V : Product  Inputs=5
  Mx : Selector  InputPortWidth=3  Indices=[1]
  My : Selector  InputPortWidth=3  Indices=[2]
  Mz : Selector  InputPortWidth=3  Indices=[3]
  OrbitalVelocity : Subsystem
  Rotation1 : Subsystem
  Rotation2 : Subsystem
  Rotation3 : Subsystem
  ShiftCg : Sum
  SwitchFx : Switch  Criteria=u2 > Threshold
  SwitchFz : Switch  Criteria=u2 > Threshold
  Terminator : Terminator
  Terminator1 : Terminator
  Ux : Selector  InputPortWidth=3  Indices=[1]
  Uy : Selector  InputPortWidth=3  Indices=[2]
  Uz : Selector  InputPortWidth=3  Indices=[3]
  V-H : Abs
  V-V : Abs
  V^2-H : Product
  V^2-V : Product
  Vel-sl : Selector  InputPortWidth=6  Indices=[1 2 3]
  "Vel-sr " : Selector  InputPortWidth=6  Indices=[4 5 6]
  VelDiff-H : Sum  Inputs=+-
  VelDiff-V : Sum  Inputs=+-
  Zshift : Selector  InputPortWidth=3  Indices=[3]
  abs-Area : Abs
  "dot{U}x" : Selector  InputPortWidth=3  Indices=[1]
  "dot{U}y" : Selector  InputPortWidth=3  Indices=[2]
  "dot{U}z" : Selector  InputPortWidth=3  Indices=[3]
  "dot{w} x r2" : vrlib/Utilities/Cross Product
  half : Constant  Value=1/2
  r x 3x1 : Product  Multiplication=Matrix(*)
  r x 3x2 : Product  Multiplication=Matrix(*)
  r x 3x3 : Product  Multiplication=Matrix(*)
  "r_{cg} x F" : vrlib/Utilities/Cross Product
  rot1 : Selector  InputPortWidth=3  Indices=[1]
  rot2 : Selector  InputPortWidth=3  Indices=[2]
  rot3 : Selector  InputPortWidth=3  Indices=[3]
  w x r : vrlib/Utilities/Cross Product
  w x w x r : vrlib/Utilities/Cross Product
  Force : Outport  PortDimensions=[1 6]  ConcatenationDimension=1
  wires:
  Vel/1 -> Vel-sl/1, "Vel-sr "/1
  w x r/1 -> Add Vel/2, w x w x r/2
  w x w x r/1 -> Add Accel/1
  "Vel-sr "/1 -> w x w x r/1, w x r/1
  r/1 -> r x 3x3/1, "dot{w} x r2"/2, w x r/2
  Accel/1 -> Accel-sl/1, Accel-sr/1
  Accel-sr/1 -> "dot{w} x r2"/1
  "dot{w} x r2"/1 -> Add Accel/2
  Accel-sl/1 -> Add Accel/3
  Add Accel/1 -> "dot{U}z"/1, "dot{U}y"/1, "dot{U}x"/1
  Vel-sl/1 -> Add Vel/1
  Disp/1 -> Disp-sl/1, Disp-sr/1
  Disp-sr/1 -> rot3/1, rot2/1, rot1/1
  rot3/1 -> Rotation2/3(rot3), Rotation1/3(rot3)
  rot1/1 -> Rotation3/1(rot1), Rotation2/1(rot1), Rotation1/1(rot1)
  rot2/1 -> Rotation3/2(rot2), Rotation2/2(rot2), Rotation1/2(rot2)
  Rotation2/1(rot[2,1-3]) -> 3x3/2
  Rotation1/1(rot[1,1-3]) -> 3x3/1
  Rotation3/1(rot[3,1-3]) -> 3x3/3
  r x 3x3/1 -> "r_{cg} x F"/1, ShiftCg/1
  Disp-sl/1 -> ShiftCg/2
  ShiftCg/1 -> Zshift/1, OrbitalVelocity/1(Disp)
  "dot{U}y"/1 -> Terminator/1
  "dot{U}x"/1 -> AccelDiff-H/2
  OrbitalVelocity/3(H-A) -> Fx-AFK/1, AccelDiff-H/1
  "dot{U}z"/1 -> AccelDiff-V/2
  Add Vel/1 -> Uy/1, Uz/1, Ux/1
  Uy/1 -> Terminator1/1
  Ux/1 -> VelDiff-H/2
  Uz/1 -> VelDiff-V/2
  OrbitalVelocity/1(H-V) -> VelDiff-H/1
  OrbitalVelocity/2(V-V) -> VelDiff-V/1
  V-V/1 -> V^2-V/2
  VelDiff-V/1 -> V-V/1, V^2-V/1
  V^2-H/1 -> Fx-V/1
  half/1 -> Fz-V/2, Fx-V/2
  Density/1 -> Fx-AFK/3, Fz-AFK/3, Fz-A/3, Fx-A/2, Fz-V/3, Fx-V/3
  V^2-V/1 -> Fz-V/1
  AccelDiff-H/1 -> Fx-A/1
  Vol/1 -> Fz-AFK/2, Fx-AFK/2, Fz-A/2, Fx-A/3
  AccelDiff-V/1 -> Fz-A/1
  OrbitalVelocity/4(V-A) -> Fz-AFK/1, AccelDiff-V/1
  Fx-V/1 -> Fx-Sum/1
  Fx-A/1 -> Fx-Sum/2
  Fx-AFK/1 -> Fx-Sum/3
  Fz-V/1 -> Fz-Sum/1
  Fz-A/1 -> Fz-Sum/2
  Fz-AFK/1 -> Fz-Sum/3
  Fy-Sum/1 -> SwitchFx/1, ForceCom/2, SwitchFz/1, Fout/2
  "r_{cg} x F"/1 -> Mz/1, My/1, Mx/1
  Mx/1 -> Fout/4
  My/1 -> Fout/5
  Mz/1 -> Fout/6
  3x3/1 -> A x 3x3/2, r x 3x3/2, r x 3x2/2, r x 3x1/2
  V-H/1 -> V^2-H/1
  VelDiff-H/1 -> V-H/1, V^2-H/2
  Zshift/1 -> SwitchFz/2, SwitchFx/2
  SwitchFz/1 -> Fout/3, ForceCom/3
  SwitchFx/1 -> Fout/1, ForceCom/1
  Fx-Sum/1 -> SwitchFx/3
  Fz-Sum/1 -> SwitchFz/3
  Az/1 -> Fz-V/5
  A/1 -> A x 3x3/1
  Ax/1 -> Fx-V/5
  Cdx/1 -> Fx-V/4
  Cdz/1 -> Fz-V/4
  A x 3x3/1 -> abs-Area/1
  abs-Area/1 -> Az/1, Ax/1
  ForceCom/1 -> "r_{cg} x F"/2
  Fout/1 -> Force/1
  Caz/1 -> Fz-A/4
  Cax/1 -> Fx-A/4
  Cd/1 -> r x 3x1/1
  r x 3x1/1 -> Cdz/1, Cdx/1
  Ca/1 -> r x 3x2/1
  r x 3x2/1 -> Caz/1, Cax/1

== system wecModel_Morrison_Heave_091514/Sphere/Wave Diffraction and Excitation Force Calculation/Iregular Wave Excitation Force/For Each Subsystem ==
  wave spectrum : Inport  Partition=on  PartitionDimension=1  PartitionWidth=1
  wave freq : Inport  Port=2  Partition=on  PartitionDimension=1  PartitionWidth=1
  wave fExt re : Inport  Port=3  Partition=on  PartitionDimension=1  PartitionWidth=1
  wave fExt im : Inport  Port=4  Partition=on  PartitionDimension=1  PartitionWidth=1
  Time : Inport  Port=5  Partition=off
  dw : Inport  Port=6  Partition=off
  phaseRand : Inport  Port=7  Partition=on  PartitionDimension=1  PartitionWidth=1
  Add : Sum  Inputs=+-
  Add2 : Sum
  Cos Wave Function : Sin  TimeSource=Use external signal  Phase=pi/2  SampleTime=0
  Divide : Product  Inputs=***
  Divide1 : Product  Inputs=***
  Divide2 : Product  Inputs=**
  For Each : ForEach  DisableCoverage=on  IndexMode=One-based
  Sin Wave Function : Sin  TimeSource=Use external signal  SampleTime=0
  Sqrt : Sqrt  SaturateOnIntegerOverflow=on
  wxt : Product  Inputs=**
  Out1 : Outport  ConcatenationDimension=1
  wires:
  Divide1/1 -> Add/2
  Divide/1 -> Add/1
  wave fExt im/1 -> Divide1/3
  Sin Wave Function/1 -> Divide1/2
  wave freq/1 -> wxt/1
  wave fExt re/1 -> Divide/3
  Cos Wave Function/1 -> Divide/2
  Add/1 -> Out1/1
  Time/1 -> wxt/2
  wave spectrum/1 -> Divide2/1
  dw/1 -> Divide2/2
  Divide2/1 -> Sqrt/1
  Sqrt/1 -> Divide1/1, Divide/1
  wxt/1 -> Add2/1
  phaseRand/1 -> Add2/2
  Add2/1 -> Sin Wave Function/1, Cos Wave Function/1

== system wecModel_Morrison_Heave_091514/Sphere/ViscousDampingForceCalculation/IrregularWaves/MorrisonElements/MorisonElementIrregular ==
  Disp : Inport  Partition=off
  waves.kirr : Inport  Port=2  Partition=on  PartitionDimension=1  PartitionWidth=1
  waves.w : Inport  Port=3  Partition=on  PartitionDimension=1  PartitionWidth=1
  waves.A : Inport  Port=4  Partition=on  PartitionDimension=1  PartitionWidth=1
  waves.RandPhase : Inport  Port=5  Partition=on  PartitionDimension=1  PartitionWidth=1
  For Each : ForEach  DisableCoverage=on  IndexMode=One-based
  OrbitalVelocity : Subsystem
  H-V : Outport  ConcatenationDimension=1
  V-V : Outport  Port=2  ConcatenationDimension=1
  H-A : Outport  Port=3  ConcatenationDimension=1
  V-A : Outport  Port=4  ConcatenationDimension=1
  wires:
  Disp/1 -> OrbitalVelocity/1(Disp)
  waves.kirr/1 -> OrbitalVelocity/2(WaveNumber)
  waves.w/1 -> OrbitalVelocity/3(WaveFreq)
  waves.A/1 -> OrbitalVelocity/4(WaveAmp)
  waves.RandPhase/1 -> OrbitalVelocity/5(RandPhase)
  OrbitalVelocity/1(H-V) -> H-V/1
  OrbitalVelocity/2(V-V) -> V-V/1
  OrbitalVelocity/3(H-A) -> H-A/1
  OrbitalVelocity/4(V-A) -> V-A/1

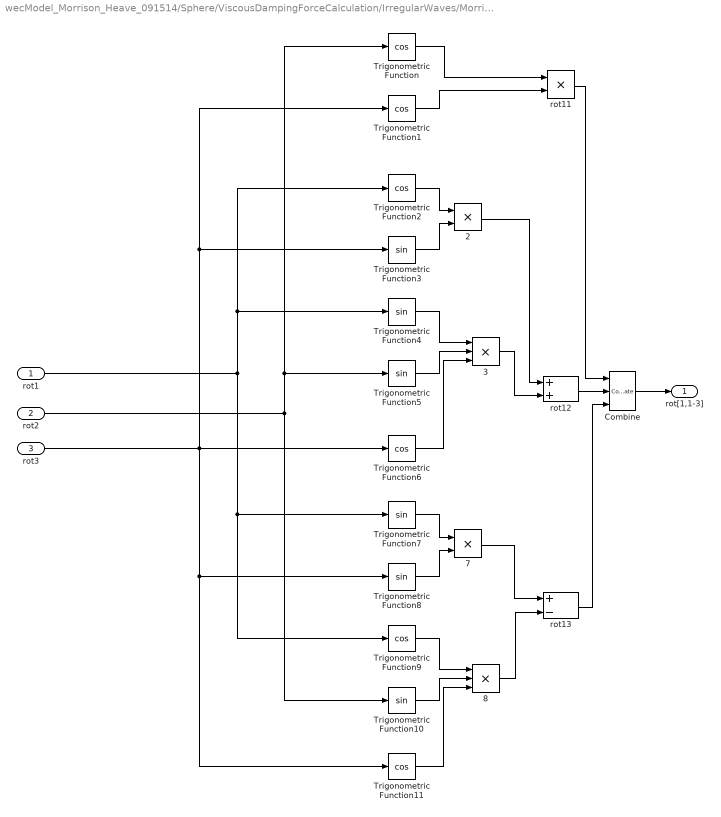
== system wecModel_Morrison_Heave_091514/Sphere/ViscousDampingForceCalculation/IrregularWaves/MorrisonElements/Rotation1 ==
  rot1 : Inport
  rot2 : Inport  Port=2
  rot3 : Inport  Port=3
  2 : Product
  3 : Product  Inputs=3
  7 : Product
  8 : Product  Inputs=3
  Combine : Concatenate  NumInputs=3  Mode=Multidimensional array  ConcatenateDimension=2
  Trigonometric Function{,1..2,6,9,11} (6 alike) : Trigonometry  Operator=cos
  Trigonometric Function{3..5,7..8,10} (6 alike) : Trigonometry
  rot11 : Product
  rot12 : Sum
  rot13 : Sum  Inputs=+-
  rot[1,1-3] : Outport
  wires:
  Trigonometric Function/1 -> rot11/1
  Trigonometric Function1/1 -> rot11/2
  rot11/1 -> Combine/1
  Trigonometric Function2/1 -> 2/1
  Trigonometric Function3/1 -> 2/2
  Trigonometric Function4/1 -> 3/1
  Trigonometric Function5/1 -> 3/2
  Trigonometric Function6/1 -> 3/3
  2/1 -> rot12/1
  3/1 -> rot12/2
  rot12/1 -> Combine/2
  Combine/1 -> rot[1,1-3]/1
  rot2/1 -> Trigonometric Function/1, Trigonometric Function5/1, Trigonometric Function10/1
  rot3/1 -> Trigonometric Function1/1, Trigonometric Function3/1, Trigonometric Function6/1, Trigonometric Function11/1, Trigonometric Function8/1
  rot1/1 -> Trigonometric Function2/1, Trigonometric Function4/1, Trigonometric Function9/1, Trigonometric Function7/1
  Trigonometric Function7/1 -> 7/1
  Trigonometric Function8/1 -> 7/2
  Trigonometric Function9/1 -> 8/1
  Trigonometric Function10/1 -> 8/2
  Trigonometric Function11/1 -> 8/3
  7/1 -> rot13/1
  8/1 -> rot13/2
  rot13/1 -> Combine/3

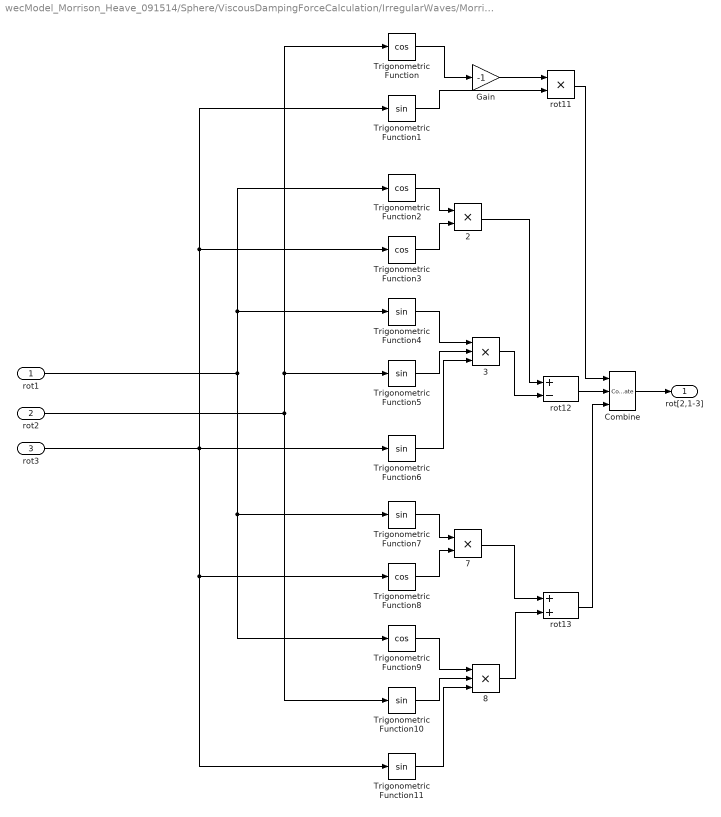
== system wecModel_Morrison_Heave_091514/Sphere/ViscousDampingForceCalculation/IrregularWaves/MorrisonElements/Rotation2 ==
  rot1 : Inport
  rot2 : Inport  Port=2
  rot3 : Inport  Port=3
  2 : Product
  3 : Product  Inputs=3
  7 : Product
  8 : Product  Inputs=3
  Combine : Concatenate  NumInputs=3  Mode=Multidimensional array  ConcatenateDimension=2
  Gain : Gain  Gain=-1
  Trigonometric Function{,2..3,8..9} (5 alike) : Trigonometry  Operator=cos
  Trigonometric Function{1,4..7,10..11} (7 alike) : Trigonometry
  rot11 : Product
  rot12 : Sum  Inputs=+-
  rot13 : Sum
  rot[2,1-3] : Outport
  wires:
  Trigonometric Function/1 -> Gain/1
  Trigonometric Function1/1 -> rot11/2
  rot11/1 -> Combine/1
  Trigonometric Function2/1 -> 2/1
  Trigonometric Function3/1 -> 2/2
  Trigonometric Function4/1 -> 3/1
  Trigonometric Function5/1 -> 3/2
  Trigonometric Function6/1 -> 3/3
  2/1 -> rot12/1
  3/1 -> rot12/2
  rot12/1 -> Combine/2
  Combine/1 -> rot[2,1-3]/1
  rot2/1 -> Trigonometric Function/1, Trigonometric Function5/1, Trigonometric Function10/1
  rot3/1 -> Trigonometric Function1/1, Trigonometric Function3/1, Trigonometric Function6/1, Trigonometric Function11/1, Trigonometric Function8/1
  rot1/1 -> Trigonometric Function2/1, Trigonometric Function4/1, Trigonometric Function9/1, Trigonometric Function7/1
  Trigonometric Function7/1 -> 7/1
  Trigonometric Function8/1 -> 7/2
  Trigonometric Function9/1 -> 8/1
  Trigonometric Function10/1 -> 8/2
  Trigonometric Function11/1 -> 8/3
  7/1 -> rot13/1
  8/1 -> rot13/2
  rot13/1 -> Combine/3
  Gain/1 -> rot11/1

== system wecModel_Morrison_Heave_091514/Sphere/ViscousDampingForceCalculation/IrregularWaves/MorrisonElements/Rotation3 ==
  rot1 : Inport
  rot2 : Inport  Port=2
  2 : Product
  7 : Product
  Combine : Concatenate  NumInputs=3  Mode=Multidimensional array  ConcatenateDimension=2
  Gain1 : Gain  Gain=-1
  TrigFun1 : Trigonometry
  TrigFun2 : Trigonometry
  TrigFun3 : Trigonometry  Operator=cos
  TrigFun4 : Trigonometry  Operator=cos
  TrigFun5 : Trigonometry  Operator=cos
  rot[3,1-3] : Outport
  wires:
  TrigFun1/1 -> Combine/1
  TrigFun3/1 -> 2/2
  2/1 -> Combine/2
  Combine/1 -> rot[3,1-3]/1
  rot2/1 -> TrigFun5/1, TrigFun3/1, TrigFun1/1
  TrigFun4/1 -> 7/1
  TrigFun5/1 -> 7/2
  rot1/1 -> TrigFun2/1, TrigFun4/1
  7/1 -> Combine/3
  TrigFun2/1 -> Gain1/1
  Gain1/1 -> 2/1

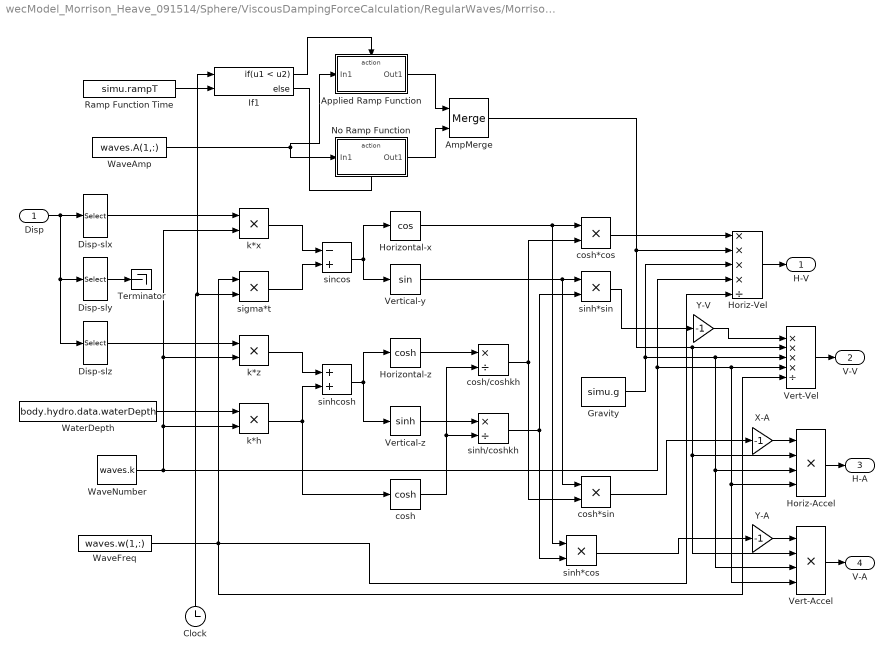
== system wecModel_Morrison_Heave_091514/Sphere/ViscousDampingForceCalculation/RegularWaves/MorrisonElements/OrbitalVelocity ==
  Disp : Inport
  AmpMerge : Merge
  Applied Ramp Function : Subsystem  TreatAsAtomicUnit=on
  Clock : Clock
  Disp-slx : Selector  InputPortWidth=3  Indices=[1]
  Disp-sly : Selector  InputPortWidth=3  Indices=[2]
  Disp-slz : Selector  InputPortWidth=3  Indices=[3]
  Gravity : Constant  Value=simu.g
  Horiz-Accel : Product  Inputs=****
  Horiz-Vel : Product  Inputs=****/
  Horizontal-x : Trigonometry  Operator=cos
  Horizontal-z : Trigonometry  Operator=cosh
  If1 : If  NumInputs=2  IfExpression=u1 < u2
  No Ramp Function : Subsystem  TreatAsAtomicUnit=on
  Ramp Function Time : Constant  Value=simu.rampT
  Terminator : Terminator
  Vert-Accel : Product  Inputs=****
  Vert-Vel : Product  Inputs=****/
  Vertical-y : Trigonometry
  Vertical-z : Trigonometry  Operator=sinh
  WaterDepth : Constant  Value=body.hydro.data.waterDepth
  WaveAmp : Constant  Value=waves.A(1,:)
  WaveFreq : Constant  Value=waves.w(1,:)
  WaveNumber : Constant  Value=waves.k
  X-A : Gain  Gain=-1
  Y-A : Gain  Gain=-1
  Y-V : Gain  Gain=-1
  cosh : Trigonometry  Operator=cosh
  cosh*cos : Product  Inputs=**
  cosh*sin : Product  Inputs=**
  cosh/coshkh : Product  Inputs=*/
  k*h : Product
  k*x : Product
  k*z : Product
  sigma*t : Product
  sincos : Sum  Inputs=-+
  sinh*cos : Product  Inputs=**
  sinh*sin : Product  Inputs=**
  sinh/coshkh : Product  Inputs=*/
  sinhcosh : Sum
  H-V : Outport
  V-V : Outport  Port=2
  H-A : Outport  Port=3
  V-A : Outport  Port=4
  wires:
  Disp/1 -> Disp-slz/1, Disp-sly/1, Disp-slx/1
  Disp-slx/1 -> k*x/1
  WaveNumber/1 -> k*h/2, k*z/2, k*x/2, Vert-Vel/4, Vert-Accel/4, Horiz-Accel/4, Horiz-Vel/4
  WaterDepth/1 -> k*h/1
  sigma*t/1 -> sincos/2
  k*x/1 -> sincos/1
  sincos/1 -> Vertical-y/1, Horizontal-x/1
  k*z/1 -> sinhcosh/1
  k*h/1 -> cosh/1, sinhcosh/2
  sinhcosh/1 -> Vertical-z/1, Horizontal-z/1
  Horizontal-z/1 -> cosh/coshkh/1
  cosh/1 -> sinh/coshkh/2, cosh/coshkh/2
  Vertical-z/1 -> sinh/coshkh/1
  Vertical-y/1 -> sinh*sin/1, cosh*sin/1
  sinh/coshkh/1 -> sinh*cos/2, sinh*sin/2
  Horizontal-x/1 -> cosh*cos/1, sinh*cos/1
  cosh/coshkh/1 -> cosh*cos/2, cosh*sin/2
  Disp-sly/1 -> Terminator/1
  cosh*cos/1 -> Horiz-Vel/1
  AmpMerge/1 -> Vert-Vel/2, Vert-Accel/2, Horiz-Accel/2, Horiz-Vel/2
  Gravity/1 -> Vert-Vel/3, Vert-Accel/3, Horiz-Accel/3, Horiz-Vel/3
  sinh*sin/1 -> Y-V/1
  Y-V/1 -> Vert-Vel/1
  X-A/1 -> Horiz-Accel/1
  Y-A/1 -> Vert-Accel/1
  Horiz-Vel/1 -> H-V/1
  Vert-Vel/1 -> V-V/1
  Horiz-Accel/1 -> H-A/1
  Vert-Accel/1 -> V-A/1
  cosh*sin/1 -> X-A/1
  sinh*cos/1 -> Y-A/1
  Ramp Function Time/1 -> If1/2
  If1/2 -> No Ramp Function/Action
  If1/1 -> Applied Ramp Function/Action
  Clock/1 -> sigma*t/2, If1/1
  No Ramp Function/1(Out1) -> AmpMerge/2
  Applied Ramp Function/1(Out1) -> AmpMerge/1
  Disp-slz/1 -> k*z/1
  WaveFreq/1 -> sigma*t/1, Horiz-Vel/5, Vert-Vel/5
  WaveAmp/1 -> Applied Ramp Function/1(In1), No Ramp Function/1(In1)
